simulink subsystem "dummy_control_subsys"  (R2022b)
settings: Solver=VariableStepAuto  StartTime=0.0  StopTime=10.0  RelTol=1e-3
settings Model: Creator=emu  LastModifiedBy=emu

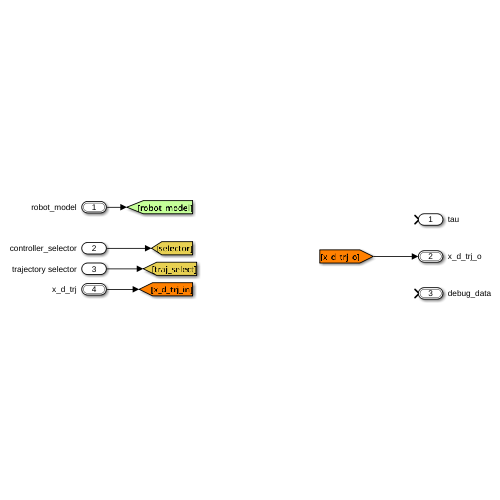
[thumbnail: Simulink's stored preview of the top-level diagram]
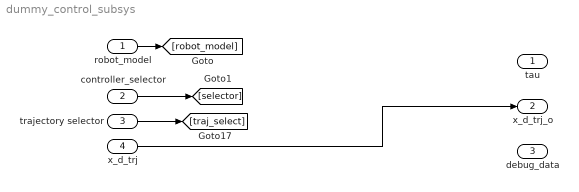
== system dummy_control_subsys ==
  robot_model : Inport  OutDataTypeStr=Bus: robot_model
  controller_selector : Inport  Port=2
  trajectory selector : Inport  Port=3
  x_d_trj : Inport  Port=4  OutDataTypeStr=Bus: x_d
  tau : Outport
  x_d_trj_o : Outport  Port=2  OutDataTypeStr=Bus: x_d
  debug_data : Outport  Port=3  OutDataTypeStr=Bus: debug_data_bus
  wires:
  controller_selector/1 -> [selector]
  robot_model/1 -> [robot_model]
  trajectory selector/1 -> [traj_select]
  x_d_trj/1 -> x_d_trj_o/1
